simulink model "requirements01"  (R2024a)
settings: Solver=FixedStepAuto  StartTime=0.0  StopTime=100  FixedStep=0.1  RelTol=1e-3
settings Model: Creator=amir  LastModifiedBy=amir

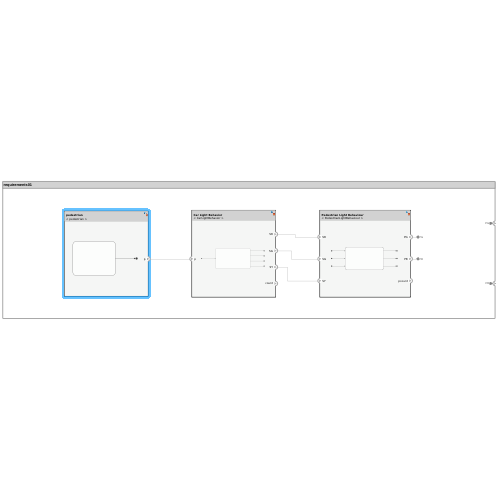
[thumbnail: Simulink's stored preview of the top-level diagram]
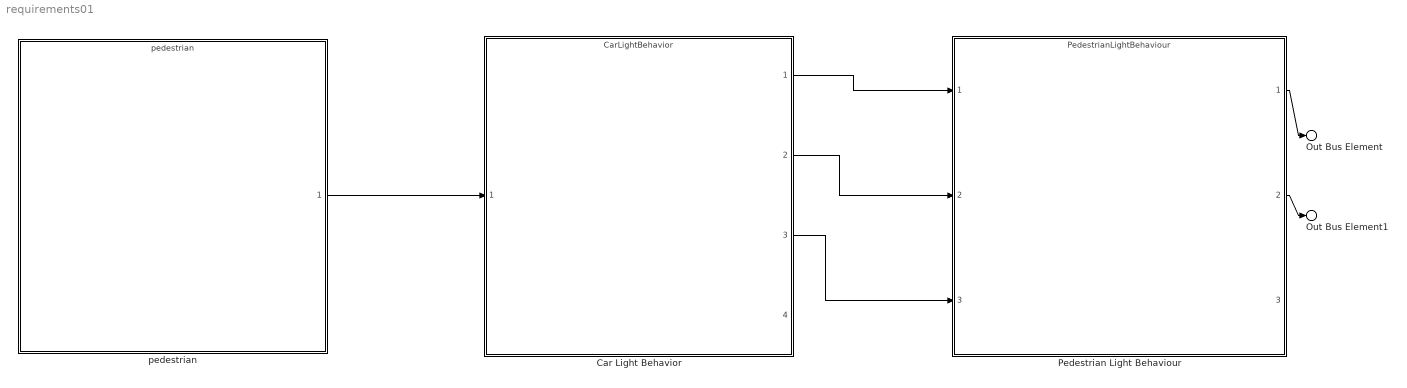
== system requirements01 ==
  Car Light Behavior : ModelReference  ModelNameDialog=CarLightBehavior  SimulationMode=Normal  ModelReferenceVersion=1.4
      settings: PortSchema="{\"entries\":[{\"content\":{\"headerSize\":38,\"margin\":15,\"minimumSpacing\":25,\"sides\":[{\"content\":{\"connectorIds\":[\"In1\"]},\"type\":\"ConnectorPlacement.EquallySpacedRectSide\",\"uuid\":\"48726829-d86d-461c-b3f1-a9b4bbd6b695\"},{\"content\":{\"connectorIds\":[\"Out1\",\"Out2\",\"Out3\",\"Out4\"],\"side\":\"RIGHT\"},\"type\":\"ConnectorPlacement.EquallySpacedRectSide\",\"uuid\":\"4ff77f49-fdf8-4120-97ad-bb22e2b131c5\"},{\"content\":{\"side\":\"TOP\"},\"type\":\"ConnectorPlacement.EquallySpacedRectSide\",\"uuid\":\"b9798bfe-0ecf-4d40-a284-8acf4e1ad550\"}]},\"type\":\"ConnectorPlacement.EquallySpacedConnector\",\"uuid\":\"dfbb9b41-0bc8-4650-9c2d-4ffd36c28d79\"}],\"packageUris\":[\"http://schema.mathworks.com/mf0/Connector/R2020b\"],\"version\":\"1.0\"}"
  Pedestrian Light Behaviour : ModelReference  ModelNameDialog=PedestrianLightBehaviour  SimulationMode=Normal  ModelReferenceVersion=1.3
      settings: PortSchema="{\"entries\":[{\"content\":{\"headerSize\":38,\"margin\":15,\"minimumSpacing\":25,\"sides\":[{\"content\":{\"connectorIds\":[\"In1\",\"In2\",\"In3\"]},\"type\":\"ConnectorPlacement.EquallySpacedRectSide\",\"uuid\":\"48726829-d86d-461c-b3f1-a9b4bbd6b695\"},{\"content\":{\"connectorIds\":[\"Out1\",\"Out2\",\"Out3\"],\"side\":\"RIGHT\"},\"type\":\"ConnectorPlacement.EquallySpacedRectSide\",\"uuid\":\"4ff77f49-fdf8-4120-97ad-bb22e2b131c5\"},{\"content\":{\"side\":\"TOP\"},\"type\":\"ConnectorPlacement.EquallySpacedRectSide\",\"uuid\":\"b9798bfe-0ecf-4d40-a284-8acf4e1ad550\"}]},\"type\":\"ConnectorPlacement.EquallySpacedConnector\",\"uuid\":\"dfbb9b41-0bc8-4650-9c2d-4ffd36c28d79\"}],\"packageUris\":[\"http://schema.mathworks.com/mf0/Connector/R2020b\"],\"version\":\"1.0\"}"
  pedestrian : ModelReference  ModelNameDialog=pedestrian.slx  SimulationMode=Normal  ModelReferenceVersion=1.3
      settings: PortSchema="{\"entries\":[{\"content\":{\"headerSize\":38,\"margin\":15,\"minimumSpacing\":25,\"sides\":[{\"content\":{},\"type\":\"ConnectorPlacement.EquallySpacedRectSide\",\"uuid\":\"48726829-d86d-461c-b3f1-a9b4bbd6b695\"},{\"content\":{\"connectorIds\":[\"Out1\"],\"side\":\"RIGHT\"},\"type\":\"ConnectorPlacement.EquallySpacedRectSide\",\"uuid\":\"4ff77f49-fdf8-4120-97ad-bb22e2b131c5\"},{\"content\":{\"side\":\"TOP\"},\"type\":\"ConnectorPlacement.EquallySpacedRectSide\",\"uuid\":\"b9798bfe-0ecf-4d40-a284-8acf4e1ad550\"}]},\"type\":\"ConnectorPlacement.EquallySpacedConnector\",\"uuid\":\"dfbb9b41-0bc8-4650-9c2d-4ffd36c28d79\"}],\"packageUris\":[\"http://schema.mathworks.com/mf0/Connector/R2020b\"],\"version\":\"1.0\"}"
  Out Bus Element : Outport  PortName=PG
  Out Bus Element1 : Outport  Port=2  PortName=PR
  wires:
  Car Light Behavior/1 -> Pedestrian Light Behaviour/1
  Car Light Behavior/2 -> Pedestrian Light Behaviour/2
  Car Light Behavior/3 -> Pedestrian Light Behaviour/3
  Pedestrian Light Behaviour/1 -> Out Bus Element/1
  Pedestrian Light Behaviour/2 -> Out Bus Element1/1
  pedestrian/1 -> Car Light Behavior/1
